simulink library "Simple_lib"  (R2018b)
settings: Solver=ode45  StartTime=0.0  StopTime=10.0  RelTol=1e-3  EnableMultiTasking=on
undefined symbols (not defined in the file or in its folder): Acceptance, beta, C, C_J, C_P, c_wall, dGain, DiscIntNeverNeededParam, Duplex, Electrical_lib, grab, h_fe, i, i3, K_T, Kman, KmanCE, mu_s, n_rev, R_arm, Simplex, systemTs, tau_0, TinIC, Ts, w_0, wallMass, Watch_lib
libraries: $bdroot x407, PlantUtilityBlockset_lib x30, peGeneralControl x22, simulink x11
(part 9 of 14)

== system Simple_lib/Hydraulic/Pump ==
  P : Inport
  w : Inport  Port=2
  T : Inport  Port=3
  Area : Gain
  Area1 : Gain  Gain=-1
  Area3 : Gain  Gain=-1
  Bus Creator : BusCreator  Inputs=2
  Bus Creator1 : BusCreator  Inputs=2
  Bus Selector : BusSelector  OutputSignals=p,T
  Bus Selector1 : BusSelector  OutputSignals=T,p
  PushBack : PlantUtilityBlockset_lib/Utility/Push  SystemSampleTime=-1
  PushBack1 : PlantUtilityBlockset_lib/Utility/Push  SystemSampleTime=-1
  PushBack2 : PlantUtilityBlockset_lib/Utility/Push  SystemSampleTime=-1
  Q : Constant  Value=[100 100 100 100 100 100]
  Q1 : Constant  Value=[100 100 100 100 100 100]
  Sum : Sum  Inputs=+|+
  Terminator : Terminator
  Terminator1 : Terminator
  VolPerRad : Gain
  wires:
  Bus Creator1/1 -> PushBack1/2
  Q1/1 -> Bus Creator1/1  "Q"
  Q/1 -> Bus Creator/2  "Q"
  Bus Creator/1 -> PushBack/2
  Bus Selector1/1 -> Terminator1/1  "<T>"
  PushBack1/1 -> Bus Selector1/1
  PushBack/1 -> Bus Selector/1
  T/1 -> PushBack1/1
  Bus Selector/2 -> Terminator/1  "<T>"
  P/1 -> PushBack/1
  VolPerRad/1 -> Area3/1, Bus Creator1/2  "q"
  Area3/1 -> Bus Creator/1  "q"
  PushBack2/1 -> VolPerRad/1
  Area1/1 -> Sum/2
  Area/1 -> PushBack2/2
  Sum/1 -> Area/1
  Bus Selector1/2 -> Area1/1  "<p>"
  Bus Selector/1 -> Sum/1  "<p>"
  w/1 -> PushBack2/1

== system Simple_lib/Hydraulic/Quadratic Heat Pipe ==
  pT_in : Inport
  Display1 : Display
  Gain : Gain  Gain=-1
  Gain1 : Gain  Gain=1e3
  I1O1BoxIIValveCannelloniHydro6 : Scope
  Product : Product  Inputs=***//  RndMeth=Zero
  Pull : Subsystem  Tag=Electrical  AncestorBlock=PlantUtilityBlockset_lib/Utility/Pull  InitFcn=initDuplex
      mask Display:
      | color('white')
      | plot([0 3], [2 2])
      | plot([0 3], [-2 -2])
      | color('black')
      | 
      | plot([0 1 1], [0 0 0.4])
      | plot([1 1 3], [0.6 1 1])
      | plot([1 3 2 1 0 2], [0.6 0.6 0.4 0.6 0.4 0.4])
      | patch([0 2 1],[0.4 0.4 0.6],[0,0,0])
      | plot([3 2 2], [1 1 0.6])
      | plot([2 2 3], [0.4 -1 -1])
  Push : Subsystem  AncestorBlock=PlantUtilityBlockset_lib/Utility/Push  InitFcn=initSimplex
      mask Display:
      | color('white')
      | plot([0 3], [2 2])
      | plot([0 3], [-2 -2])
      | color('black')
      | 
      | plot([0 2 2 3], [1 1 0 0])
      | plot([1 3 2 1 0 2], [0.6 0.6 0.4 0.6 0.4 0.4])
      | patch([1 3 2],[0.6 0.6 0.4],[0,0,0])
      | plot([0 1 1], [1 1 0.6])
      | plot([1 1 0], [0.4 -1 -1])
  Sign : Signum
  Sum : Sum  Inputs=|++
  area : Gain  Gain=0.1
  area offset : Constant  Value=0.1
  pT_out : Outport
  wires:
  Push/1(OutPot) -> Sum/1
  Sum/1 -> Pull/1(InPot)
  Gain/1 -> Sum/2
  Product/1 -> Gain1/1
  Pull/2(OutFlow) -> Display1/1, I1O1BoxIIValveCannelloniHydro6/1, Product/1, Push/2(InFlow), Sign/1, Product/3
  area offset/1 -> area/1
  Sign/1 -> Product/2
  Gain1/1 -> Gain/1
  area/1 -> Product/5, Product/4
  Pull/1(OutPot) -> pT_out/1
  pT_in/1 -> Push/1(InPot)

== system Simple_lib/Hydraulic/Quadratic Pipe ==
  pT_in : Inport
  Display1 : Display
  Gain : Gain  Gain=-1
  Gain1 : Gain  Gain=1e3
  I1O1BoxIIValveCannelloniHydro6 : Scope
  Product : Product  Inputs=***//  RndMeth=Zero
  Pull : Subsystem  Tag=Electrical  AncestorBlock=PlantUtilityBlockset_lib/Utility/Pull  InitFcn=initDuplex
      mask Display:
      | color('white')
      | plot([0 3], [2 2])
      | plot([0 3], [-2 -2])
      | color('black')
      | 
      | plot([0 1 1], [0 0 0.4])
      | plot([1 1 3], [0.6 1 1])
      | plot([1 3 2 1 0 2], [0.6 0.6 0.4 0.6 0.4 0.4])
      | patch([0 2 1],[0.4 0.4 0.6],[0,0,0])
      | plot([3 2 2], [1 1 0.6])
      | plot([2 2 3], [0.4 -1 -1])
  Push : Subsystem  AncestorBlock=PlantUtilityBlockset_lib/Utility/Push  InitFcn=initSimplex
      mask Display:
      | color('white')
      | plot([0 3], [2 2])
      | plot([0 3], [-2 -2])
      | color('black')
      | 
      | plot([0 2 2 3], [1 1 0 0])
      | plot([1 3 2 1 0 2], [0.6 0.6 0.4 0.6 0.4 0.4])
      | patch([1 3 2],[0.6 0.6 0.4],[0,0,0])
      | plot([0 1 1], [1 1 0.6])
      | plot([1 1 0], [0.4 -1 -1])
  Sign : Signum
  Sum : Sum  Inputs=|++
  area : Gain  Gain=0.1
  area offset : Constant  Value=0.1
  pT_out : Outport
  wires:
  Push/1(OutPot) -> Sum/1
  Sum/1 -> Pull/1(InPot)
  Gain/1 -> Sum/2
  Product/1 -> Gain1/1
  Pull/2(OutFlow) -> Display1/1, I1O1BoxIIValveCannelloniHydro6/1, Product/1, Push/2(InFlow), Sign/1, Product/3
  area offset/1 -> area/1
  Sign/1 -> Product/2
  Gain1/1 -> Gain/1
  area/1 -> Product/5, Product/4
  Pull/1(OutPot) -> pT_out/1
  pT_in/1 -> Push/1(InPot)

== system Simple_lib/Hydraulic/Tank ==
  Ambient Pressure : Constant  Value=1e5
  Duplex : PlantUtilityBlockset_lib/Utility/Pull  Tag=Electrical  SystemSampleTime=-1
  Terminator : Terminator
  Out1 : Outport
  wires:
  Duplex/1 -> Out1/1
  Ambient Pressure/1 -> Duplex/1
  Duplex/2 -> Terminator/1

== system Simple_lib/Hydraulic/Water-Glycol Heat Exchanger ==
  pTSea_in : Inport
  pTGly_in : Inport  Port=2
  Pipe1 : Subsystem  AncestorBlock=PlantUtilityBlockset_lib/Hydraulic/Quadratic Pipe  InitFcn=bond
      mask Display:
      | plot([-1:0.2:1], [1 .7 .5 .4 .35 .32 .35 .4 .5 .7 1])
      | plot([-1:0.2:1], -[1 .7 .5 .4 .35 .32 .35 .4 .5 .7 1])
  Pipe2 : Subsystem  AncestorBlock=PlantUtilityBlockset_lib/Hydraulic/Quadratic Pipe  InitFcn=bond
      mask Display:
      | plot([-1:0.2:1], [1 .7 .5 .4 .35 .32 .35 .4 .5 .7 1])
      | plot([-1:0.2:1], -[1 .7 .5 .4 .35 .32 .35 .4 .5 .7 1])
  pTSea_out : Outport
  pTGly_out : Outport  Port=2
  wires:
  Pipe1/1(pT_out) -> pTSea_out/1
  Pipe2/1(pT_out) -> pTGly_out/1
  pTGly_in/1 -> Pipe2/1(pT_in)
  pTSea_in/1 -> Pipe1/1(pT_in)

== system Simple_lib/Hydraulic/X Heat Exchanger ==
  in1 : Inport
  in2 : Inport  Port=2
  Pipe1 : Subsystem  AncestorBlock=PlantUtilityBlockset_lib/Hydraulic/Quadratic Pipe
      mask Display:
      | plot([-1:0.2:1], [1 .7 .5 .4 .35 .32 .35 .4 .5 .7 1])
      | plot([-1:0.2:1], -[1 .7 .5 .4 .35 .32 .35 .4 .5 .7 1])
  Pipe2 : Subsystem  AncestorBlock=PlantUtilityBlockset_lib/Hydraulic/Quadratic Pipe
      mask Display:
      | plot([-1:0.2:1], [1 .7 .5 .4 .35 .32 .35 .4 .5 .7 1])
      | plot([-1:0.2:1], -[1 .7 .5 .4 .35 .32 .35 .4 .5 .7 1])
  out1 : Outport
  out2 : Outport  Port=2
  wires:
  Pipe1/1(pT_out) -> out1/1
  Pipe2/1(pT_out) -> out2/1
  in2/1 -> Pipe2/1(pT_in)
  in1/1 -> Pipe1/1(pT_in)

== system Simple_lib/Junkyard/CinWall ==
  C : Subsystem  AncestorBlock=PlantUtilityBlockset_lib/Electrical/C  mask{C=wallMass*c_wall}
      mask prompts: C "Capacitance"
      mask Display:
      | color('white')
      | plot([-1 1 1 -1 -1], [-1 -1 1 1 -1])
      | color('black')
      | plot([1.0 1.8 1.8 1.0], [0 .1 -.1 0])
      | plot([-1 -1], [-1 1])
      | plot([1 1], [-1 1])
  Gnd : Subsystem  AncestorBlock=PlantUtilityBlockset_lib/Electrical/Gnd
      mask Display:
      | color('white')
      | plot([-1 1 1 -1 -1], [-1 -1 1 1 -1])
      | 
      | color('black')
      | plot([1.0 1.18 1.18 1.0], [0 .15 -.15 0])
      | 
      | plot([-0.4 -0.4],[-1 1])
      | plot([-0.6 -0.6], [-0.6 0.6])
      | plot([-0.8 -0.8],[-0.2 0.2])
      | 
      | plot([-0.4 1],[0 0])
  Out1 : Outport
  wires:
  C/1(Out1) -> Out1/1
  Gnd/1(Out1) -> C/1(In1)

== system Simple_lib/Junkyard/Conventional Flow  ==
  In1 : Inport
  Out1 : Outport
  wires:
  In1/1 -> Out1/1

== system Simple_lib/Junkyard/R13 ==
  In1 : Inport
  Duplex : Subsystem  Tag=Electrical  AncestorBlock=PlantUtilityBlockset_lib/Utility/Duplex  InitFcn=initDuplex
      mask Display:
      | color('white')
      | plot([0 3], [2 2])
      | plot([0 3], [-2 -2])
      | color('black')
      | 
      | plot([0 1 1], [0 0 0.4])
      | plot([1 1 3], [0.6 1 1])
      | plot([1 3 2 1 0 2], [0.6 0.6 0.4 0.6 0.4 0.4])
      | patch([0 2 1],[0.4 0.4 0.6],[0,0,0])
      | plot([3 2 2], [1 1 0.6])
      | plot([2 2 3], [0.4 -1 -1])
  Simplex : Subsystem  Tag=Electrical  AncestorBlock=PlantUtilityBlockset_lib/Utility/Simplex  InitFcn=initSimplex
      mask Display:
      | color('white')
      | plot([0 3], [2 2])
      | plot([0 3], [-2 -2])
      | color('black')
      | 
      | plot([0 2 2 3], [1 1 0 0])
      | plot([1 3 2 1 0 2], [0.6 0.6 0.4 0.6 0.4 0.4])
      | patch([1 3 2],[0.6 0.6 0.4],[0,0,0])
      | plot([0 1 1], [1 1 0.6])
      | plot([1 1 0], [0.4 -1 -1])
  Sum : Sum  Inputs=|++
  resistance : Gain  Gain=R
  Out1 : Outport
  wires:
  In1/1 -> Simplex/1(InPot)
  Duplex/1(OutPot) -> Out1/1
  Duplex/2(OutFlow) -> Simplex/2(InFlow), resistance/1
  Simplex/1(OutPot) -> Sum/1
  resistance/1 -> Sum/2
  Sum/1 -> Duplex/1(InPot)

== system Simple_lib/Junkyard/R17 ==
  In1 : Inport
  In2 : Inport  Port=2
  1/R1 : Gain  Gain=-1
  1/R2 : Gain  Gain=-1
  Discrete-Time Integrator1 : DiscreteIntegrator  gainval=1/10/Ts  SampleTime=Ts  ICPrevOutput=DiscIntNeverNeededParam  ICPrevScaledInput=DiscIntNeverNeededParam
  Simplex : Subsystem  Tag=Electrical  AncestorBlock=PlantUtilityBlockset_lib/Utility/Simplex  InitFcn=initSimplex
      mask Display:
      | color('white')
      | plot([0 3], [2 2])
      | plot([0 3], [-2 -2])
      | color('black')
      | 
      | plot([0 2 2 3], [1 1 0 0])
      | plot([1 3 2 1 0 2], [0.6 0.6 0.4 0.6 0.4 0.4])
      | patch([1 3 2],[0.6 0.6 0.4],[0,0,0])
      | plot([0 1 1], [1 1 0.6])
      | plot([1 1 0], [0.4 -1 -1])
  Simplex1 : Subsystem  Tag=Electrical  AncestorBlock=PlantUtilityBlockset_lib/Utility/Simplex  InitFcn=initSimplex
      mask Display:
      | color('white')
      | plot([0 3], [2 2])
      | plot([0 3], [-2 -2])
      | color('black')
      | 
      | plot([0 2 2 3], [1 1 0 0])
      | plot([1 3 2 1 0 2], [0.6 0.6 0.4 0.6 0.4 0.4])
      | patch([1 3 2],[0.6 0.6 0.4],[0,0,0])
      | plot([0 1 1], [1 1 0.6])
      | plot([1 1 0], [0.4 -1 -1])
  Sum : Sum  Inputs=+|+
  Sum1 : Sum  Inputs=|+-
  conductance : Gain  Gain=1/R
  wires:
  Discrete-Time Integrator1/1 -> Sum1/2, 1/R1/1, Simplex/2(InFlow)
  Sum1/1 -> Discrete-Time Integrator1/1
  1/R1/1 -> Simplex1/2(InFlow)
  Simplex1/1(OutPot) -> Sum/2
  In2/1 -> Simplex1/1(InPot)
  Sum/1 -> conductance/1
  1/R2/1 -> Sum/1
  Simplex/1(OutPot) -> 1/R2/1
  In1/1 -> Simplex/1(InPot)
  conductance/1 -> Sum1/1

== system Simple_lib/Junkyard/ThermoMeter ==
  In : Inport
  Ground : Ground
  PushBack : Subsystem  AncestorBlock=PlantUtilityBlockset_lib/Utility/Push  InitFcn=initSimplex
      mask Display:
      | color('white')
      | plot([0 3], [2 2])
      | plot([0 3], [-2 -2])
      | color('black')
      | 
      | plot([0 2 2 3], [1 1 0 0])
      | plot([1 3 2 1 0 2], [0.6 0.6 0.4 0.6 0.4 0.4])
      | patch([1 3 2],[0.6 0.6 0.4],[0,0,0])
      | plot([0 1 1], [1 1 0.6])
      | plot([1 1 0], [0.4 -1 -1])
  T : Outport
  wires:
  In/1 -> PushBack/1(InPot)
  PushBack/1(OutPot) -> T/1
  Ground/1 -> PushBack/2(InFlow)

== system Simple_lib/Junkyard/Unconventional Flow ==
  In1 : Inport
  Out1 : Outport
  wires:
  In1/1 -> Out1/1

== system Simple_lib/Magnetic/BiGain ==
  In1 : Inport
  Bus Creator1 : BusCreator  Inputs=2
  Bus Selector : BusSelector  OutputSignals=F,M
  _in : $bdroot/Translational/_in  Level=v  Flow=F
  _out : $bdroot/Translational/_out  Tag=Electrical  Level=v  Flow=F
  k_flow : Gain  Gain=k_flow
  k_flow1 : Gain  Gain=k_flow
  k_flow2 : Gain  Gain=k_flow
  k_level : Gain  Gain=k_level
  Out1 : Outport
  wires:
  _out/1 -> Out1/1
  _in/1 -> k_level/1
  In1/1 -> _in/1
  k_level/1 -> _out/1
  _out/2 -> Bus Selector/1
  k_flow/1 -> Bus Creator1/1  "F"
  Bus Selector/2 -> k_flow2/1  "<M>"
  Bus Selector/1 -> k_flow/1  "<F>"
  Bus Creator1/1 -> _in/2
  k_flow2/1 -> k_flow1/1  "M"
  k_flow1/1 -> Bus Creator1/2  "M"

== system Simple_lib/Magnetic/Core ==
  + : Inport
  - : Inport  Port=2
  1/R3 : Gain  Gain=-1
  Bus Creator : BusCreator  Inputs=2
  Bus Creator1 : BusCreator  Inputs=2
  Derivative : Derivative
  Ground : Ground
  Ground1 : Ground
  M : Gain  Gain=b
  Sum : Sum  Inputs=+|-
  _neg : $bdroot/Magnetic/_in  Level=MMF  Flow=Phi
  _pos : $bdroot/Magnetic/_in  Level=MMF  Flow=Phi
  wires:
  1/R3/1 -> Bus Creator/1  "dPhi"
  Sum/1 -> Derivative/1
  Derivative/1 -> M/1  "dI1"
  -/1 -> _neg/1
  _pos/1 -> Sum/1  "I1"
  _neg/1 -> Sum/2  "I2"
  M/1 -> 1/R3/1, Bus Creator1/1  "dPhi"
  Bus Creator1/1 -> _pos/2
  Ground/1 -> Bus Creator/2  "MagneticInertia"
  +/1 -> _pos/1  "mmf"
  Bus Creator/1 -> _neg/2
  Ground1/1 -> Bus Creator1/2  "MagneticInertia"

== system Simple_lib/Magnetic/Core_old ==
  + : Inport
  - : Inport  Port=2
  1/R1 : Gain  Gain=b
  1/R3 : Gain  Gain=b
  Bus Creator : BusCreator  Inputs=2
  Bus Creator1 : BusCreator  Inputs=2
  Discrete Derivative : simulink/Discrete/Discrete Derivative  gainval=1  ICPrevScaledInput=0.0  OutMin=[]  OutMax=[]  OutDataType=fixdt(1, 16)  OutScaling=2^-10  DoSatur=off
  Discrete Derivative1 : simulink/Discrete/Discrete Derivative  gainval=1  ICPrevScaledInput=0.0  OutMin=[]  OutMax=[]  OutDataType=fixdt(1, 16)  OutScaling=2^-10  DoSatur=off
  Ground : Ground
  Ground1 : Ground
  _neg : $bdroot/Magnetic/_in  Level=MMF  Flow=Phi
  _pos : $bdroot/Magnetic/_in  Level=MMF  Flow=Phi
  wires:
  Discrete Derivative1/1 -> 1/R1/1  "dI1"
  Discrete Derivative/1 -> 1/R3/1  "dI2"
  -/1 -> _neg/1
  1/R1/1 -> Bus Creator/1  "dPhi"
  _pos/1 -> Discrete Derivative1/1  "I1"
  _neg/1 -> Discrete Derivative/1  "I2"
  1/R3/1 -> Bus Creator1/1  "dPhi"
  Bus Creator1/1 -> _pos/2
  Ground/1 -> Bus Creator/2  "MagneticInertia"
  +/1 -> _pos/1  "mmf"
  Bus Creator/1 -> _neg/2
  Ground1/1 -> Bus Creator1/2  "MagneticInertia"

== system Simple_lib/Magnetic/Friction ==
  pos : Inport
  K : Inport  Port=2
  neg : Inport  Port=3
  1/R1 : Gain  Gain=-1
  1/R2 : Gain  Gain=-1
  1/R3 : Gain  Gain=-1
  Bus Creator : BusCreator  Inputs=2
  Bus Creator1 : BusCreator  Inputs=2
  Discrete-Time Integrator : DiscreteIntegrator  gainval=1  SampleTime=-1  ICPrevOutput=DiscIntNeverNeededParam  ICPrevScaledInput=DiscIntNeverNeededParam
  Exp : Math  SaturateOnIntegerOverflow=on
  Gain : Gain  Gain=-1/2
  Ground : Ground
  Multiply : Product
  Multiply1 : Product  Inputs=**//
  Multiply2 : Product  Inputs=**/
  Sum : Sum  Inputs=+|+
  Sum1 : Sum  Inputs=|++
  _neg : $bdroot/Translational/_in  Level=v  Flow=F
  _pos : $bdroot/Translational/_in  Level=v  Flow=F
  friction : Trigonometry  Operator=tanh
  grab : Gain  Gain=grab
  sigma : Constant  Value=s
  synche : Gain  Gain=Ki/sqrt(2*pi)
  wires:
  synche/1 -> Sum1/2
  friction/1 -> Multiply/2
  Sum/1 -> grab/1
  Discrete-Time Integrator/1 -> synche/1
  Sum1/1 -> friction/1
  Gain/1 -> Exp/1
  sigma/1 -> Multiply1/3, Multiply1/4, Multiply2/3
  Multiply2/1 -> Discrete-Time Integrator/1
  Exp/1 -> Multiply2/2
  Multiply1/1 -> Gain/1
  _neg/1 -> 1/R3/1
  Multiply/1 -> 1/R2/1
  _pos/1 -> Sum/1
  grab/1 -> Multiply2/1, Multiply1/2, Multiply1/1, Sum1/1
  pos/1 -> _pos/1
  neg/1 -> _neg/1
  K/1 -> Multiply/1
  Bus Creator1/1 -> _pos/2
  1/R2/1 -> Bus Creator1/1, 1/R1/1  "F"
  Bus Creator/1 -> _neg/2
  Ground/1 -> Bus Creator1/2, Bus Creator/2  "M"
  1/R1/1 -> Bus Creator/1  "F"
  1/R3/1 -> Sum/2

== system Simple_lib/Magnetic/Sink ==
  In1 : Inport
  Bus Creator : BusCreator  Inputs=2
  Constant : Constant  Value=m
  Ground : Ground
  Terminator : Terminator
  _at : $bdroot/Translational/_in  Level=v  Flow=F
  wires:
  Bus Creator/1 -> _at/2
  In1/1 -> _at/1
  _at/1 -> Terminator/1
  Ground/1 -> Bus Creator/1  "F"
  Constant/1 -> Bus Creator/2  "M"

== system Simple_lib/Magnetic/Source ==
  note: Newton's law for all the applied torques (real parts) and the inertials (imaginary parts).
  Bus Selector : BusSelector  OutputSignals=F,M
  Constant : Constant  Value=m
  Discrete-Time Integrator1 : DiscreteIntegrator  gainval=1  InitialCondition=v_0  SampleTime=-1  ICPrevOutput=DiscIntNeverNeededParam  ICPrevScaledInput=DiscIntNeverNeededParam
  Multiply : Product  Inputs=*/
  Saturation : Saturate  UpperLimit=inf  LowerLimit=Ts*1e-3
  Sum : Sum  Inputs=|++
  _at : $bdroot/Translational/_out  Tag=Electrical  Level=v  Flow=F
  Out1 : Outport
  wires:
  _at/1 -> Out1/1
  Multiply/1 -> Discrete-Time Integrator1/1
  _at/2 -> Bus Selector/1
  Bus Selector/1 -> Multiply/1  "<F>"
  Bus Selector/2 -> Sum/1  "<M>"
  Sum/1 -> Saturation/1
  Constant/1 -> Sum/2
  Discrete-Time Integrator1/1 -> _at/1
  Saturation/1 -> Multiply/2

== system Simple_lib/Magnetic/SpringDamper ==
  in : Inport
  Damping : $bdroot/Translational/Damping  b=b_damper
  Source1 : $bdroot/Translational/Source  m=m_out  v_0=v_0
      settings: AttributesFormatString=%<m> kg
  Stiffness : $bdroot/Translational/Stiffness  k_spring=k_spring  s_0=s_0  I_spring=m_split  b_series=b_spring
  Terminator : Terminator
  out : Outport
  wires:
  in/1 -> Damping/1, Stiffness/1
  Source1/1 -> Damping/2, Stiffness/2, out/1
  Stiffness/1 -> Terminator/1

== system Simple_lib/Magnetic/Stiffness ==
  + : Inport
  - : Inport  Port=2
  Bus Creator : BusCreator  Inputs=2
  Bus Creator1 : BusCreator  Inputs=2
  Constant : Constant  Value=I_spring/2
  Constant1 : Constant  Value=I_spring/2
  Discrete-Time Integrator1 : DiscreteIntegrator  gainval=1  InitialCondition=s_0  SampleTime=-1  ICPrevOutput=DiscIntNeverNeededParam  ICPrevScaledInput=DiscIntNeverNeededParam
  Gain : Gain  Gain=-k_spring
  Gain1 : Gain  Gain=k_spring
  Gain2 : Gain  Gain=2/b_series
  Gain3 : Gain  Gain=2/b_series
  Sum : Sum  Inputs=+|-
  Sum1 : Sum  Inputs=++|
  Sum2 : Sum  Inputs=++|
  _neg : $bdroot/Translational/_in  Level=v  Flow=F
  _pos : $bdroot/Translational/_in  Level=v  Flow=F
  cmp : Outport
  wires:
  _neg/1 -> Sum2/1
  -/1 -> _neg/1
  Sum/1 -> Discrete-Time Integrator1/1
  _pos/1 -> Sum1/1
  +/1 -> _pos/1
  Bus Creator1/1 -> _pos/2
  Bus Creator/1 -> _neg/2
  Discrete-Time Integrator1/1 -> cmp/1, Gain1/1, Gain/1  "cmp"
  Constant/1 -> Bus Creator1/2  "M"
  Constant1/1 -> Bus Creator/1  "M"
  Sum2/1 -> Sum/2
  Sum1/1 -> Sum/1
  Gain/1 -> Gain2/1, Bus Creator1/1  "F"
  Gain1/1 -> Bus Creator/2, Gain3/1  "F"
  Gain2/1 -> Sum1/2
  Gain3/1 -> Sum2/2

== system Simple_lib/Magnetic/_in ==
  note: {\bf\_in - wraps up the {\itInflow} block}
      |
      | The init function {\itinit_in} sets up the logging of the level and flow names.
  in : Inport
  back : Inport  Port=2
  Bus Selector : BusSelector  OutputSignals=dPhi,MagneticInertia
  Inflow : $bdroot/Utility/Inflow  SystemSampleTime=-1
  Mux : Mux  Inputs=2
  out : Outport
  wires:
  in/1 -> Inflow/1  "MMF"
  back/1 -> Bus Selector/1
  Bus Selector/2 -> Mux/2  "<MagneticInertia>"
  Bus Selector/1 -> Mux/1  "<dPhi>"
  Inflow/1 -> out/1
  Mux/1 -> Inflow/2

== system Simple_lib/Magnetic/_out ==
  note: {\bf\_out - buses out and logs the signals from the generic {\itOutflow} block}
      |
      | The init function {\itinit\_out} sets up the logging.
  in : Inport  Tag=NOFLUX
  Bus Creator : BusCreator  Inputs=2
  Constant : Constant  Value=[0;0]
  Demux : Demux  Outputs=2
  Outflow : $bdroot/Utility/Outflow  Tag=Electrical  SystemSampleTime=-1
  Sum : Sum  Inputs=|++
  Sum1 : Sum  Inputs=+  CollapseMode=Specified dimension  CollapseDim=2
  out : Outport
  backs : Outport  Tag=NOFLUX  Port=2
  wires:
  Outflow/1 -> out/1
  Sum1/1 -> Sum/1
  Demux/1 -> Bus Creator/1  "dPhi"
  Bus Creator/1 -> backs/1
  Outflow/2 -> Sum1/1
  in/1 -> Outflow/1  "MMF"
  Demux/2 -> Bus Creator/2  "MagneticInertia"
  Constant/1 -> Sum/2
  Sum/1 -> Demux/1

== system Simple_lib/Magnetic/magR ==
  + : Inport
  - : Inport  Port=2
  1/R3 : Gain  Gain=b
  Bus Creator : BusCreator  Inputs=2
  Bus Creator1 : BusCreator  Inputs=2
  Discrete Derivative : simulink/Discrete/Discrete Derivative  Commented=through  gainval=1  ICPrevScaledInput=0.0  OutMin=[]  OutMax=[]  OutDataType=fixdt(1, 16)  OutScaling=2^-10  DoSatur=off
  Gain1 : Gain  Gain=-1
  Ground : Ground
  Ground1 : Ground
  Sum : Sum  Inputs=+|-
  _neg : $bdroot/Magnetic/_in  Level=MMF  Flow=Phi
  _pos : $bdroot/Magnetic/_in  Level=MMF  Flow=Phi
  wires:
  Discrete Derivative/1 -> 1/R3/1
  -/1 -> _neg/1
  _neg/1 -> Sum/2
  1/R3/1 -> Bus Creator/1, Gain1/1  "dPhi"
  Bus Creator1/1 -> _pos/2
  Ground/1 -> Bus Creator/2  "MagneticInertia"
  +/1 -> _pos/1  "mmf"
  _pos/1 -> Sum/1
  Sum/1 -> Discrete Derivative/1
  Bus Creator/1 -> _neg/2
  Ground1/1 -> Bus Creator1/2  "MagneticInertia"
  Gain1/1 -> Bus Creator1/1  "dPhi"

== system Simple_lib/Rotational/BiGain ==
  In1 : Inport
  Bus Creator1 : BusCreator  Inputs=3
  Bus Selector : BusSelector  OutputSignals=tau,c,J
  _in : $bdroot/Rotational/_in  Level=w  Flow=tau
  _out : $bdroot/Rotational/_out  Tag=Electrical  Level=w  Flow=tau
  k_flow{1..5} (5 alike) : Gain  Gain=k_flow
  k_pot : Gain  Gain=k_flow
  Out1 : Outport
  wires:
  _out/1 -> Out1/1
  _in/1 -> k_pot/1
  In1/1 -> _in/1
  Bus Creator1/1 -> _in/2
  k_pot/1 -> _out/1
  _out/2 -> Bus Selector/1
  Bus Selector/1 -> k_flow1/1  "<tau>"
  Bus Selector/3 -> k_flow3/1  "<J>"
  k_flow1/1 -> Bus Creator1/1  "tau"
  k_flow2/1 -> Bus Creator1/3  "J"
  k_flow3/1 -> k_flow2/1  "M"
  Bus Selector/2 -> k_flow5/1  "<c>"
  k_flow4/1 -> Bus Creator1/2  "c"
  k_flow5/1 -> k_flow4/1

== system Simple_lib/Rotational/Damping ==
  + : Inport
  - : Inport  Port=2
  1/R3 : Gain  Gain=b
  Bus Creator : BusCreator  Inputs=3
  Bus Creator1 : BusCreator  Inputs=3
  Constant : Constant  Value=b
  Gain1 : Gain  Gain=-1
  Gain2 : Gain  Gain=-1
  Ground : Ground
  Sum : Sum  Inputs=+|+
  _neg : $bdroot/Rotational/_in  Level=w  Flow=tau
  _pos : $bdroot/Rotational/_in  Level=w  Flow=tau
  wires:
  Constant/1 -> Bus Creator1/2, Bus Creator/2  "c"
  _neg/1 -> Gain2/1
  1/R3/1 -> Bus Creator1/1, Gain1/1  "tau"
  Bus Creator1/1 -> _pos/2
  +/1 -> _pos/1
  _pos/1 -> Sum/1
  Sum/1 -> 1/R3/1
  -/1 -> _neg/1
  Bus Creator/1 -> _neg/2
  Ground/1 -> Bus Creator1/3, Bus Creator/1  "J"
  Gain1/1 -> Bus Creator/3  "tau"
  Gain2/1 -> Sum/2  "tau"

== system Simple_lib/Rotational/Friction ==
  pos : Inport
  K : Inport  Port=2
  neg : Inport  Port=3
  1/R1 : Gain  Gain=-1
  Bus Creator : BusCreator  Inputs=3
  Bus Creator1 : BusCreator  Inputs=3
  Calculate Slip : Subsystem
  Derivative : Subsystem
  Gaussian Spring : Subsystem
  Ground : Ground
  Multiply : Product
  Sum1 : Sum  Inputs=|++
  _neg : $bdroot/Rotational/_in  Level=w  Flow=tau
  _pos : $bdroot/Rotational/_in  Level=w  Flow=tau
  wires:
  _neg/1 -> Calculate Slip/2(w_neg)  "w_neg"
  _pos/1 -> Calculate Slip/1(w_pos)  "w_pos"
  Calculate Slip/1(slip) -> Derivative/2(x), Gaussian Spring/1(slip), Sum1/1
  Derivative/1(dy/dx) -> Bus Creator1/2, Bus Creator/2  "c"
  Gaussian Spring/1(tau) -> Sum1/2
  1/R1/1 -> Bus Creator1/3  "tau"
  Sum1/1 -> Multiply/2
  neg/1 -> _neg/1
  pos/1 -> _pos/1
  K/1 -> Multiply/1
  Bus Creator1/1 -> _neg/2
  Multiply/1 -> Derivative/1(y), Bus Creator/1, 1/R1/1  "tau"
  Bus Creator/1 -> _pos/2
  Ground/1 -> Bus Creator1/1, Bus Creator/3  "J"

== system Simple_lib/Rotational/Inertia ==
  In1 : Inport
  Bus Creator : BusCreator  Inputs=3
  Constant : Constant  Value=I
  Ground : Ground
  Ground1 : Ground
  Terminator : Terminator
  _at : $bdroot/Rotational/_in  Level=w  Flow=tau
  wires:
  Ground1/1 -> Bus Creator/2  "c"
  Bus Creator/1 -> _at/2
  In1/1 -> _at/1
  _at/1 -> Terminator/1
  Ground/1 -> Bus Creator/1  "tau"
  Constant/1 -> Bus Creator/3  "J"

== system Simple_lib/Rotational/Lump ==
  note: Newton's law for all the applied torques and the inertials.
      | If the inertia sum is too small to give sensible results we approximate from the damping coefficients.
      | If that is really small we saturate at J = e-12 Nm2.
      | We also saturate the overall acceleration to configurable parameter max_accel.
  Abs2 : Abs
  Abs3 : Abs
  Bus Selector : BusSelector  OutputSignals=tau,c,J
  Constant : Constant  Value=w_0
  Constant1 : Constant  Value=1/2
  Ground : Ground
  Integrator (Discrete or Continuous) : peGeneralControl/Integrator (Discrete or Continuous)  LabelModeActiveChoice=Discrete  ExternalReset=level  LimitType=Anti-windup  B=inf  A=-inf  Ts=-1
  Max1 : MinMax  Function=max  Inputs=2
  Momentum outflow decelerates : Gain  Gain=-1
  Multiply : Product  Inputs=*/
  Multiply1 : Product  Inputs=3
  Multiply2 : Product
  Saturation : Saturate  UpperLimit=inf  LowerLimit=1e-12
      settings: AttributesFormatString=|
      | %<UpperLimit>
      | %<LowerLimit>
  Saturation3 : Saturate  UpperLimit=max_accel  LowerLimit=-max_accel
      settings: AttributesFormatString=|
      | %<UpperLimit>
      | %<LowerLimit>
  Terminator : Terminator
  Terminator1 : Terminator
  Weighted Sample Time1 : SampleTimeMath  TsampMathOp=*  weightValue=1
  _off : $bdroot/Rotational/_out  Tag=Electrical  Level=w  Flow=tau
  Out1 : Outport
  wires:
  Constant1/1 -> Multiply1/2
  Multiply1/1 -> Terminator1/1  "energy"
  Multiply2/1 -> Terminator/1, Multiply1/3  "conserved_quantity"
  Saturation3/1 -> Integrator (Discrete or Continuous)/1  "dw_sat"
  Abs3/1 -> Max1/1  "JestPos"
  Abs2/1 -> Max1/2  "Jpos"
  Bus Selector/2 -> Weighted Sample Time1/1  "<c>"
  Max1/1 -> Saturation/1  "Jeff"
  Weighted Sample Time1/1 -> Abs3/1  "Jest"
  _off/1 -> Out1/1
  Multiply/1 -> Saturation3/1  "dw"
  _off/2 -> Bus Selector/1
  Bus Selector/1 -> Momentum outflow decelerates/1  "<tau>"
  Bus Selector/3 -> Abs2/1  "<J>"
  Integrator (Discrete or Continuous)/1 -> _off/1, Multiply1/1, Multiply2/1  "w"
  Saturation/1 -> Multiply/2, Multiply2/2  "Jeff_sat"
  Constant/1 -> Integrator (Discrete or Continuous)/3
  Ground/1 -> Integrator (Discrete or Continuous)/2
  Momentum outflow decelerates/1 -> Multiply/1

== system Simple_lib/Rotational/M1 ==
  In1 : Inport
  _at : $bdroot/Rotational/_out  Tag=Electrical  Level=w  Flow=tau
  _thru : $bdroot/Rotational/_in  Level=w  Flow=tau
  Out1 : Outport
  wires:
  _at/1 -> Out1/1
  In1/1 -> _thru/1
  _thru/1 -> _at/1
  _at/2 -> _thru/2

== system Simple_lib/Rotational/NonLinear Compliance ==
  + : Inport
  - : Inport  Port=2
  1-D Lookup Table : Lookup_n-D  NumberOfTableDimensions=1  BreakpointsForDimension1=[-5:5]*10  Table=[100 10 1 0 0 0 0 0 1 10 100]  InternalRulePriority=Speed  RndMeth=Simplest  InputSameDT=on
  Bus Creator : BusCreator  Inputs=2
  Bus Creator1 : BusCreator  Inputs=2
  Constant : Constant  Value=I_spring/2
  Constant1 : Constant  Value=I_spring/2
  Discrete-Time Integrator1 : DiscreteIntegrator  gainval=1  InitialCondition=theta_0  SampleTime=-1  ICPrevOutput=DiscIntNeverNeededParam  ICPrevScaledInput=DiscIntNeverNeededParam
  Gain : Gain  Gain=-k_spring
  Gain1 : Gain  Gain=k_spring
  Gain2 : Gain  Gain=2/b_series
  Gain3 : Gain  Gain=2/b_series
  Gain4 : Gain  Gain=-1
  Sum : Sum  Inputs=+|-
  Sum1 : Sum  Inputs=++|
  Sum2 : Sum  Inputs=++|
  _neg : $bdroot/Rotational/_in  Level=w  Flow=tau
  _pos : $bdroot/Rotational/_in  Level=w  Flow=tau
  cmp : Outport
  wires:
  Gain4/1 -> cmp/1, Gain/1, Gain1/1
  1-D Lookup Table/1 -> Gain4/1
  _neg/1 -> Sum2/1
  -/1 -> _neg/1
  Sum/1 -> Discrete-Time Integrator1/1
  _pos/1 -> Sum1/1
  +/1 -> _pos/1
  Bus Creator1/1 -> _pos/2
  Bus Creator/1 -> _neg/2
  Discrete-Time Integrator1/1 -> 1-D Lookup Table/1  "cmp"
  Constant/1 -> Bus Creator1/2  "J"
  Constant1/1 -> Bus Creator/1  "J"
  Sum2/1 -> Sum/2
  Sum1/1 -> Sum/1
  Gain/1 -> Gain2/1, Bus Creator1/1  "tau"
  Gain1/1 -> Bus Creator/2, Gain3/1  "tau"
  Gain2/1 -> Sum1/2
  Gain3/1 -> Sum2/2

== system Simple_lib/Rotational/Power ==
  " " : Inport
  Bus Creator1 : BusCreator  Inputs=2
  Bus Selector : BusSelector  OutputSignals=tau,J
  Multiply : Product
  Torque_Speed : simulink/Sinks/XY Graph  Commented=on  xmin=0  xmax=200  ymin=-1  ymax=1  st=-1
  _in : $bdroot/Rotational/_in  Level=w  Flow=tau
  _out : $bdroot/Rotational/_out  Tag=Electrical  Level=w  Flow=tau
  "  " : Outport
  > : Outport  Port=2
  wires:
  Multiply/1 -> >/1
  _out/1 -> "  "/1
  " "/1 -> _in/1
  Bus Creator1/1 -> _in/2
  _in/1 -> Torque_Speed/1, _out/1, Multiply/1  "w"
  _out/2 -> Bus Selector/1
  Bus Selector/1 -> Bus Creator1/1, Torque_Speed/2, Multiply/2  "<tau>"
  Bus Selector/2 -> Bus Creator1/2  "<J>"

== system Simple_lib/Rotational/Speed ==
  w : Inport
  Terminator1 : Terminator
  _at : $bdroot/Rotational/_out  Tag=Electrical  Level=w  Flow=tau
  sys : Outport
  wires:
  w/1 -> _at/1
  _at/1 -> sys/1
  _at/2 -> Terminator1/1

== system Simple_lib/Rotational/SpringDamper ==
  in : Inport
  Damping : $bdroot/Rotational/Damping  b=b_damper
  Source : $bdroot/Rotational/Lump  w_0=w_0  max_accel=inf
  Stiffness : $bdroot/Rotational/Stiffness  k_spring=k_spring  theta_0=theta_0  I_spring=I_split  b_series=b_spring
  Terminator : Terminator
  out : Outport
  wires:
  in/1 -> Stiffness/1, Damping/1
  Source/1 -> Stiffness/2, Damping/2, out/1
  Stiffness/1 -> Terminator/1

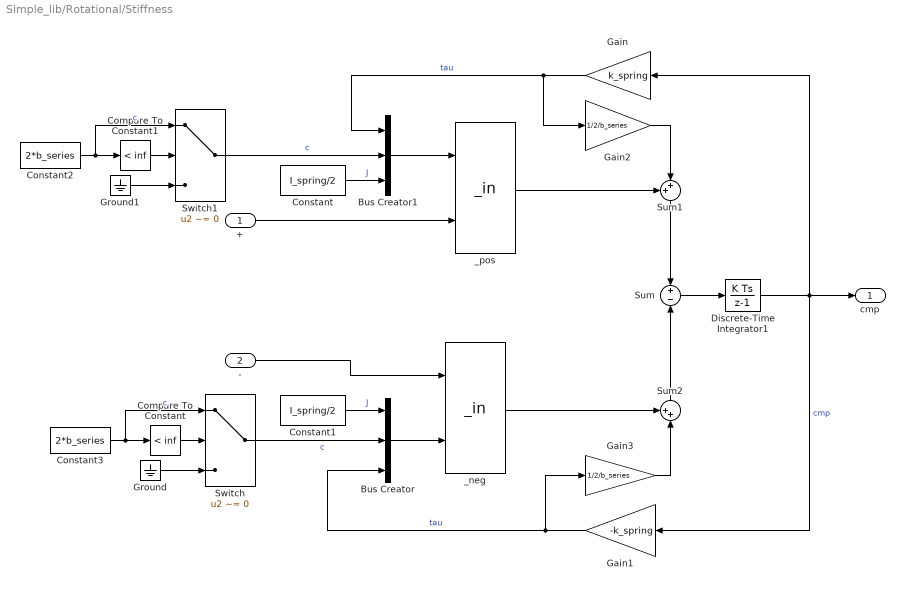
== system Simple_lib/Rotational/Stiffness ==
  + : Inport
  - : Inport  Port=2
  Bus Creator : BusCreator  Inputs=3
  Bus Creator1 : BusCreator  Inputs=3
  Compare To Constant : simulink/Logic and Bit Operations/Compare To Constant  relop=<  const=inf  OutDataTypeStr=boolean
  Compare To Constant1 : simulink/Logic and Bit Operations/Compare To Constant  relop=<  const=inf  OutDataTypeStr=boolean
  Constant : Constant  Value=I_spring/2
  Constant1 : Constant  Value=I_spring/2
  Constant2 : Constant  Value=2*b_series
  Constant3 : Constant  Value=2*b_series
  Discrete-Time Integrator1 : DiscreteIntegrator  gainval=1  InitialCondition=theta_0  SampleTime=-1  ICPrevOutput=DiscIntNeverNeededParam  ICPrevScaledInput=DiscIntNeverNeededParam
  Gain : Gain  Gain=k_spring
  Gain1 : Gain  Gain=-k_spring
  Gain2 : Gain  Gain=1/2/b_series
  Gain3 : Gain  Gain=1/2/b_series
  Ground : Ground
  Ground1 : Ground
  Sum : Sum  Inputs=+|-
  Sum1 : Sum  Inputs=++|
  Sum2 : Sum  Inputs=++|
  Switch : Switch  Criteria=u2 ~= 0
  Switch1 : Switch  Criteria=u2 ~= 0
  _neg : $bdroot/Rotational/_in  Level=w  Flow=tau
  _pos : $bdroot/Rotational/_in  Level=w  Flow=tau
  cmp : Outport
  wires:
  Constant3/1 -> Switch/1, Compare To Constant/1  "c"
  Switch1/1 -> Bus Creator1/2  "c"
  _neg/1 -> Sum2/1
  -/1 -> _neg/1
  Sum/1 -> Discrete-Time Integrator1/1
  _pos/1 -> Sum1/1
  +/1 -> _pos/1
  Bus Creator1/1 -> _pos/2
  Bus Creator/1 -> _neg/2
  Discrete-Time Integrator1/1 -> cmp/1, Gain1/1, Gain/1  "cmp"
  Constant/1 -> Bus Creator1/3  "J"
  Constant1/1 -> Bus Creator/1  "J"
  Sum2/1 -> Sum/2
  Sum1/1 -> Sum/1
  Gain/1 -> Gain2/1, Bus Creator1/1  "tau"
  Gain1/1 -> Bus Creator/3, Gain3/1  "tau"
  Gain2/1 -> Sum1/2
  Gain3/1 -> Sum2/2
  Compare To Constant/1 -> Switch/2
  Ground/1 -> Switch/3
  Switch/1 -> Bus Creator/2  "c"
  Ground1/1 -> Switch1/3
  Compare To Constant1/1 -> Switch1/2
  Constant2/1 -> Switch1/1, Compare To Constant1/1  "c"

== system Simple_lib/Rotational/Torque ==
  sys : Inport
  tau : Inport  Port=2
  Bus Creator : BusCreator  Inputs=3
  Ground : Ground
  Ground1 : Ground
  Terminator1 : Terminator
  _at : $bdroot/Rotational/_in  Level=w  Flow=tau
  wires:
  tau/1 -> Bus Creator/1  "tau"
  _at/1 -> Terminator1/1
  sys/1 -> _at/1
  Bus Creator/1 -> _at/2
  Ground/1 -> Bus Creator/3  "J"
  Ground1/1 -> Bus Creator/2  "c"

== system Simple_lib/Rotational/_in ==
  note: {\bf\_in - wraps up the {\itInflow} block}
      |
      | The init function {\itinit_in} sets up the logging of the level and flow names.
  in : Inport
  back : Inport  Port=2
  Bus Selector : BusSelector  OutputSignals=tau,c,J
  Inflow : $bdroot/Utility/Inflow  SystemSampleTime=-1
  Mux : Mux  Inputs=3
  out : Outport
  wires:
  Bus Selector/2 -> Mux/2  "<c>"
  in/1 -> Inflow/1  "w"
  back/1 -> Bus Selector/1
  Bus Selector/3 -> Mux/3  "<J>"
  Bus Selector/1 -> Mux/1  "<tau>"
  Inflow/1 -> out/1
  Mux/1 -> Inflow/2

== system Simple_lib/Rotational/_out ==
  note: {\bf\_out - buses out and logs the signals from the generic {\itOutflow} block}
      |
      | The init function {\itinit\_out} sets up the logging.
  in : Inport  Tag=NOFLUX
  Bus Creator : BusCreator  Inputs=3
  Constant : Constant  Value=[0;0;0]
  Demux : Demux  Outputs=3
  Outflow : $bdroot/Utility/Outflow  Tag=Electrical  SystemSampleTime=-1
  Sum : Sum  Inputs=|++
  Sum1 : Sum  Inputs=+  CollapseMode=Specified dimension  CollapseDim=2
  out : Outport
  backs : Outport  Tag=NOFLUX  Port=2
  wires:
  Demux/3 -> Bus Creator/3  "J"
  Outflow/1 -> out/1
  Sum1/1 -> Sum/1
  Demux/1 -> Bus Creator/1  "tau"
  Bus Creator/1 -> backs/1
  Outflow/2 -> Sum1/1
  in/1 -> Outflow/1  "w"
  Demux/2 -> Bus Creator/2  "c"
  Constant/1 -> Sum/2
  Sum/1 -> Demux/1

== system Simple_lib/Thermal/CinWall ==
  C : Subsystem  AncestorBlock=PlantUtilityBlockset_lib/Electrical/C  mask{C=wallMass*c_wall}
      mask prompts: C "Capacitance"
      mask Display:
      | color('white')
      | plot([-1 1 1 -1 -1], [-1 -1 1 1 -1])
      | color('black')
      | plot([1.0 1.8 1.8 1.0], [0 .1 -.1 0])
      | plot([-1 -1], [-1 1])
      | plot([1 1], [-1 1])
  Gnd : Subsystem  AncestorBlock=PlantUtilityBlockset_lib/Electrical/Gnd
      mask Display:
      | color('white')
      | plot([-1 1 1 -1 -1], [-1 -1 1 1 -1])
      | 
      | color('black')
      | plot([1.0 1.18 1.18 1.0], [0 .15 -.15 0])
      | 
      | plot([-0.4 -0.4],[-1 1])
      | plot([-0.6 -0.6], [-0.6 0.6])
      | plot([-0.8 -0.8],[-0.2 0.2])
      | 
      | plot([-0.4 1],[0 0])
  Out1 : Outport
  wires:
  C/1(Out1) -> Out1/1
  Gnd/1(Out1) -> C/1(In1)

== system Simple_lib/Thermal/R13 ==
  In1 : Inport
  Duplex : Subsystem  Tag=Electrical  AncestorBlock=PlantUtilityBlockset_lib/Utility/Duplex  InitFcn=initDuplex
      mask Display:
      | color('white')
      | plot([0 3], [2 2])
      | plot([0 3], [-2 -2])
      | color('black')
      | 
      | plot([0 1 1], [0 0 0.4])
      | plot([1 1 3], [0.6 1 1])
      | plot([1 3 2 1 0 2], [0.6 0.6 0.4 0.6 0.4 0.4])
      | patch([0 2 1],[0.4 0.4 0.6],[0,0,0])
      | plot([3 2 2], [1 1 0.6])
      | plot([2 2 3], [0.4 -1 -1])
  Simplex : Subsystem  Tag=Electrical  AncestorBlock=PlantUtilityBlockset_lib/Utility/Simplex  InitFcn=initSimplex
      mask Display:
      | color('white')
      | plot([0 3], [2 2])
      | plot([0 3], [-2 -2])
      | color('black')
      | 
      | plot([0 2 2 3], [1 1 0 0])
      | plot([1 3 2 1 0 2], [0.6 0.6 0.4 0.6 0.4 0.4])
      | patch([1 3 2],[0.6 0.6 0.4],[0,0,0])
      | plot([0 1 1], [1 1 0.6])
      | plot([1 1 0], [0.4 -1 -1])
  Sum : Sum  Inputs=|++
  resistance : Gain  Gain=R
  Out1 : Outport
  wires:
  In1/1 -> Simplex/1(InPot)
  Duplex/1(OutPot) -> Out1/1
  Duplex/2(OutFlow) -> Simplex/2(InFlow), resistance/1
  Simplex/1(OutPot) -> Sum/1
  resistance/1 -> Sum/2
  Sum/1 -> Duplex/1(InPot)

== system Simple_lib/Thermal/R17 ==
  In1 : Inport
  In2 : Inport  Port=2
  1/R1 : Gain  Gain=-1
  1/R2 : Gain  Gain=-1
  Discrete-Time Integrator1 : DiscreteIntegrator  gainval=1/10/Ts  SampleTime=Ts  ICPrevOutput=DiscIntNeverNeededParam  ICPrevScaledInput=DiscIntNeverNeededParam
  Simplex : Subsystem  Tag=Electrical  AncestorBlock=PlantUtilityBlockset_lib/Utility/Simplex  InitFcn=initSimplex
      mask Display:
      | color('white')
      | plot([0 3], [2 2])
      | plot([0 3], [-2 -2])
      | color('black')
      | 
      | plot([0 2 2 3], [1 1 0 0])
      | plot([1 3 2 1 0 2], [0.6 0.6 0.4 0.6 0.4 0.4])
      | patch([1 3 2],[0.6 0.6 0.4],[0,0,0])
      | plot([0 1 1], [1 1 0.6])
      | plot([1 1 0], [0.4 -1 -1])
  Simplex1 : Subsystem  Tag=Electrical  AncestorBlock=PlantUtilityBlockset_lib/Utility/Simplex  InitFcn=initSimplex
      mask Display:
      | color('white')
      | plot([0 3], [2 2])
      | plot([0 3], [-2 -2])
      | color('black')
      | 
      | plot([0 2 2 3], [1 1 0 0])
      | plot([1 3 2 1 0 2], [0.6 0.6 0.4 0.6 0.4 0.4])
      | patch([1 3 2],[0.6 0.6 0.4],[0,0,0])
      | plot([0 1 1], [1 1 0.6])
      | plot([1 1 0], [0.4 -1 -1])
  Sum : Sum  Inputs=+|+
  Sum1 : Sum  Inputs=|+-
  conductance : Gain  Gain=1/R
  wires:
  Discrete-Time Integrator1/1 -> Sum1/2, 1/R1/1, Simplex/2(InFlow)
  Sum1/1 -> Discrete-Time Integrator1/1
  1/R1/1 -> Simplex1/2(InFlow)
  Simplex1/1(OutPot) -> Sum/2
  In2/1 -> Simplex1/1(InPot)
  Sum/1 -> conductance/1
  1/R2/1 -> Sum/1
  Simplex/1(OutPot) -> 1/R2/1
  In1/1 -> Simplex/1(InPot)
  conductance/1 -> Sum1/1

== system Simple_lib/Thermal/ThermoMeter ==
  note: NOTE: Does not necessarily need Pushback
  In : Inport
  Ground : Ground
  PushBack : Subsystem  AncestorBlock=PlantUtilityBlockset_lib/Utility/Push  InitFcn=initSimplex
      mask Display:
      | color('white')
      | plot([0 3], [2 2])
      | plot([0 3], [-2 -2])
      | color('black')
      | 
      | plot([0 2 2 3], [1 1 0 0])
      | plot([1 3 2 1 0 2], [0.6 0.6 0.4 0.6 0.4 0.4])
      | patch([1 3 2],[0.6 0.6 0.4],[0,0,0])
      | plot([0 1 1], [1 1 0.6])
      | plot([1 1 0], [0.4 -1 -1])
  T : Outport
  wires:
  In/1 -> PushBack/1(InPot)
  PushBack/1(OutPot) -> T/1
  Ground/1 -> PushBack/2(InFlow)

== system Simple_lib/Translational/BiGain ==
  In1 : Inport
  Bus Creator1 : BusCreator  Inputs=2
  Bus Selector : BusSelector  OutputSignals=F,M
  _in : $bdroot/Translational/_in  Level=v  Flow=F
  _out : $bdroot/Translational/_out  Tag=Electrical  Level=v  Flow=F
  k_flow : Gain  Gain=k_flow
  k_flow1 : Gain  Gain=k_flow
  k_flow2 : Gain  Gain=k_flow
  k_level : Gain  Gain=k_level
  Out1 : Outport
  wires:
  _out/1 -> Out1/1
  _in/1 -> k_level/1
  In1/1 -> _in/1
  k_level/1 -> _out/1
  _out/2 -> Bus Selector/1
  k_flow/1 -> Bus Creator1/1  "F"
  Bus Selector/2 -> k_flow2/1  "<M>"
  Bus Selector/1 -> k_flow/1  "<F>"
  Bus Creator1/1 -> _in/2
  k_flow2/1 -> k_flow1/1  "M"
  k_flow1/1 -> Bus Creator1/2  "M"

== system Simple_lib/Translational/Damping ==
  + : Inport
  - : Inport  Port=2
  1/R3 : Gain  Gain=b
  Bus Creator : BusCreator  Inputs=2
  Bus Creator1 : BusCreator  Inputs=2
  Gain1 : Gain  Gain=-1
  Ground : Ground
  Ground1 : Ground
  Sum : Sum  Inputs=+|-
  _neg : $bdroot/Translational/_in  Level=v  Flow=F
  _pos : $bdroot/Translational/_in  Level=v  Flow=F
  wires:
  _neg/1 -> Sum/2
  1/R3/1 -> Bus Creator/1, Gain1/1  "F"
  Bus Creator1/1 -> _pos/2
  Ground/1 -> Bus Creator/2  "M"
  +/1 -> _pos/1
  _pos/1 -> Sum/1
  Sum/1 -> 1/R3/1
  -/1 -> _neg/1
  Bus Creator/1 -> _neg/2
  Ground1/1 -> Bus Creator1/2  "M"
  Gain1/1 -> Bus Creator1/1  "F"

== system Simple_lib/Translational/Friction ==
  pos : Inport
  K : Inport  Port=2
  neg : Inport  Port=3
  1/R1 : Gain  Gain=-1
  1/R2 : Gain  Gain=-1
  1/R3 : Gain  Gain=-1
  Bus Creator : BusCreator  Inputs=2
  Bus Creator1 : BusCreator  Inputs=2
  Discrete-Time Integrator : DiscreteIntegrator  gainval=1  SampleTime=-1  ICPrevOutput=DiscIntNeverNeededParam  ICPrevScaledInput=DiscIntNeverNeededParam
  Exp : Math  SaturateOnIntegerOverflow=on
  Gain : Gain  Gain=-1/2
  Ground : Ground
  Multiply : Product
  Multiply1 : Product  Inputs=**//
  Multiply2 : Product  Inputs=**/
  Sum : Sum  Inputs=+|+
  Sum1 : Sum  Inputs=|++
  _neg : $bdroot/Translational/_in  Level=v  Flow=F
  _pos : $bdroot/Translational/_in  Level=v  Flow=F
  friction : Trigonometry  Operator=tanh
  grab : Gain  Gain=grab
  sigma : Constant  Value=s
  synche : Gain  Gain=Ki/sqrt(2*pi)
  wires:
  synche/1 -> Sum1/2
  friction/1 -> Multiply/2
  Sum/1 -> grab/1
  Discrete-Time Integrator/1 -> synche/1
  Sum1/1 -> friction/1
  Gain/1 -> Exp/1
  sigma/1 -> Multiply1/3, Multiply1/4, Multiply2/3
  Multiply2/1 -> Discrete-Time Integrator/1
  Exp/1 -> Multiply2/2
  Multiply1/1 -> Gain/1
  _neg/1 -> 1/R3/1
  Multiply/1 -> 1/R2/1
  _pos/1 -> Sum/1
  grab/1 -> Multiply2/1, Multiply1/2, Multiply1/1, Sum1/1
  pos/1 -> _pos/1
  neg/1 -> _neg/1
  K/1 -> Multiply/1
  Bus Creator1/1 -> _pos/2
  1/R2/1 -> Bus Creator1/1, 1/R1/1  "F"
  Bus Creator/1 -> _neg/2
  Ground/1 -> Bus Creator1/2, Bus Creator/2  "M"
  1/R1/1 -> Bus Creator/1  "F"
  1/R3/1 -> Sum/2

== system Simple_lib/Translational/Sink ==
  In1 : Inport
  Bus Creator : BusCreator  Inputs=2
  Constant : Constant  Value=m
  Ground : Ground
  Terminator : Terminator
  _at : $bdroot/Translational/_in  Level=v  Flow=F
  wires:
  Bus Creator/1 -> _at/2
  In1/1 -> _at/1
  _at/1 -> Terminator/1
  Ground/1 -> Bus Creator/1  "F"
  Constant/1 -> Bus Creator/2  "M"

== system Simple_lib/Translational/Source ==
  note: Newton's law for all the applied torques (real parts) and the inertials (imaginary parts).
  Bus Selector : BusSelector  OutputSignals=F,M
  Constant : Constant  Value=m
  Discrete-Time Integrator1 : DiscreteIntegrator  gainval=1  InitialCondition=v_0  SampleTime=-1  ICPrevOutput=DiscIntNeverNeededParam  ICPrevScaledInput=DiscIntNeverNeededParam
  Multiply : Product  Inputs=*/
  Saturation : Saturate  UpperLimit=inf  LowerLimit=Ts*1e-3
  Sum : Sum  Inputs=|++
  _at : $bdroot/Translational/_out  Tag=Electrical  Level=v  Flow=F
  Out1 : Outport
  wires:
  _at/1 -> Out1/1
  Multiply/1 -> Discrete-Time Integrator1/1
  _at/2 -> Bus Selector/1
  Bus Selector/1 -> Multiply/1  "<F>"
  Bus Selector/2 -> Sum/1  "<M>"
  Sum/1 -> Saturation/1
  Constant/1 -> Sum/2
  Discrete-Time Integrator1/1 -> _at/1
  Saturation/1 -> Multiply/2

== system Simple_lib/Translational/SpringDamper ==
  in : Inport
  Damping : $bdroot/Translational/Damping  b=b_damper
  Source1 : $bdroot/Translational/Source  m=m_out  v_0=v_0
      settings: AttributesFormatString=%<m> kg
  Stiffness : $bdroot/Translational/Stiffness  k_spring=k_spring  s_0=s_0  I_spring=m_split  b_series=b_spring
  Terminator : Terminator
  out : Outport
  wires:
  in/1 -> Damping/1, Stiffness/1
  Source1/1 -> Damping/2, Stiffness/2, out/1
  Stiffness/1 -> Terminator/1

== system Simple_lib/Translational/Stiffness ==
  + : Inport
  - : Inport  Port=2
  Bus Creator : BusCreator  Inputs=2
  Bus Creator1 : BusCreator  Inputs=2
  Constant : Constant  Value=I_spring/2
  Constant1 : Constant  Value=I_spring/2
  Discrete-Time Integrator1 : DiscreteIntegrator  gainval=1  InitialCondition=s_0  SampleTime=-1  ICPrevOutput=DiscIntNeverNeededParam  ICPrevScaledInput=DiscIntNeverNeededParam
  Gain : Gain  Gain=-k_spring
  Gain1 : Gain  Gain=k_spring
  Gain2 : Gain  Gain=2/b_series
  Gain3 : Gain  Gain=2/b_series
  Sum : Sum  Inputs=+|-
  Sum1 : Sum  Inputs=++|
  Sum2 : Sum  Inputs=++|
  _neg : $bdroot/Translational/_in  Level=v  Flow=F
  _pos : $bdroot/Translational/_in  Level=v  Flow=F
  cmp : Outport
  wires:
  _neg/1 -> Sum2/1
  -/1 -> _neg/1
  Sum/1 -> Discrete-Time Integrator1/1
  _pos/1 -> Sum1/1
  +/1 -> _pos/1
  Bus Creator1/1 -> _pos/2
  Bus Creator/1 -> _neg/2
  Discrete-Time Integrator1/1 -> cmp/1, Gain1/1, Gain/1  "cmp"
  Constant/1 -> Bus Creator1/2  "M"
  Constant1/1 -> Bus Creator/1  "M"
  Sum2/1 -> Sum/2
  Sum1/1 -> Sum/1
  Gain/1 -> Gain2/1, Bus Creator1/1  "F"
  Gain1/1 -> Bus Creator/2, Gain3/1  "F"
  Gain2/1 -> Sum1/2
  Gain3/1 -> Sum2/2

== system Simple_lib/Translational/_in ==
  note: {\bf\_in - wraps up the {\itInflow} block}
      |
      | The init function {\itinit_in} sets up the logging of the level and flow names.
  in : Inport
  back : Inport  Port=2
  Bus Selector : BusSelector  OutputSignals=F,M
  Inflow : $bdroot/Utility/Inflow  SystemSampleTime=-1
  Mux : Mux  Inputs=2
  out : Outport
  wires:
  in/1 -> Inflow/1  "v"
  back/1 -> Bus Selector/1
  Bus Selector/2 -> Mux/2  "<M>"
  Bus Selector/1 -> Mux/1  "<F>"
  Inflow/1 -> out/1
  Mux/1 -> Inflow/2

== system Simple_lib/Translational/_out ==
  note: {\bf\_out - buses out and logs the signals from the generic {\itOutflow} block}
      |
      | The init function {\itinit\_out} sets up the logging.
  in : Inport  Tag=NOFLUX
  Bus Creator : BusCreator  Inputs=2
  Constant : Constant  Value=[0;0]
  Demux : Demux  Outputs=2
  Outflow : $bdroot/Utility/Outflow  Tag=Electrical  SystemSampleTime=-1
  Sum : Sum  Inputs=|++
  Sum1 : Sum  Inputs=+  CollapseMode=Specified dimension  CollapseDim=2
  out : Outport
  backs : Outport  Tag=NOFLUX  Port=2
  wires:
  Outflow/1 -> out/1
  Sum1/1 -> Sum/1
  Demux/1 -> Bus Creator/1  "F"
  Bus Creator/1 -> backs/1
  Outflow/2 -> Sum1/1
  in/1 -> Outflow/1  "v"
  Demux/2 -> Bus Creator/2  "M"
  Constant/1 -> Sum/2
  Sum/1 -> Demux/1

== system Simple_lib/Utility/BiGain ==
  In1 : Inport
  Duplex : $bdroot/Utility/Outflow  Tag=Electrical  SystemSampleTime=-1
  Simplex : $bdroot/Utility/Inflow  Tag=Electrical  SystemSampleTime=-1
  Sum1 : Sum  Inputs=+
  k_flow : Gain  Gain=k_flow
  k_pot : Gain  Gain=k_pot
  Out1 : Outport
  wires:
  Duplex/2 -> Sum1/1
  Duplex/1 -> Out1/1
  Simplex/1 -> k_pot/1
  In1/1 -> Simplex/1
  k_flow/1 -> Simplex/2
  k_pot/1 -> Duplex/1
  Sum1/1 -> k_flow/1

== system Simple_lib/Utility/Duplex ==
  InPot : Inport  Tag=NOFLUX
  FlowGain : Gain
  FlowSum : Sum  Inputs=3  SaturateOnIntegerOverflow=on  InputSameDT=on  OutDataTypeStr=Inherit: Same as first input
  OutPot : Outport
  OutFlow : Outport  Tag=NOFLUX  Port=2
  wires:
  [SimplexR1StatorHeatSinkInverterPFessSchematicPower] -> FlowSum/3
  [SimplexR2StatorHeatSinkInverterPFessSchematicPower] -> FlowSum/2
  [SimplexR3StatorHeatSinkInverterPFessSchematicPower] -> FlowSum/1
  FlowGain/1 -> OutFlow/1  "flow"
  InPot/1 -> OutPot/1  "pot"
  FlowSum/1 -> FlowGain/1

== system Simple_lib/Utility/DuplexSav ==
  InPot : Inport  Tag=NOFLUX
  FlowDisplay : Display
  FlowGain : Gain
  Flow_DuplexGndC0ChargingCapacitor3 : Scope
      settings: Tag=Flow
  PotDisplay : Display
  Pot_DuplexGndC0ChargingCapacitor3 : Scope
      settings: Tag=Pot
  Rate Transition : RateTransition  OutPortSampleTimeMultiple=nT  OutPortSampleTime=Ts
  OutPot : Outport
  OutFlow : Outport  Tag=NOFLUX  Port=2
  wires:
  [SimplexCC0ChargingCapacitor3] -> FlowGain/1
  FlowGain/1 -> FlowDisplay/1, OutFlow/1, Flow_DuplexGndC0ChargingCapacitor3/1
  InPot/1 -> Pot_DuplexGndC0ChargingCapacitor3/1, PotDisplay/1, Rate Transition/1
  Rate Transition/1 -> OutPot/1

== system Simple_lib/Utility/Inflow ==
  note: {\bfBack - sends a signal back using a {\itGoto} block}
      |
      | The init function {\itsmpInit} creates the Goto block with a unique name.
  in : Inport
  back : Inport  Port=2
  Terminator : Terminator
  out : Outport
  tag scope: tagInflowUtilitySimple_lib=global
  wires:
  back/1 -> [tagInflowUtilitySimple_lib]
  in/1 -> out/1
  [tagInflowUtilitySimple_lib] -> Terminator/1

== system Simple_lib/Utility/Inflow_old ==
  note: {\bfBack - sends a signal back using a {\itGoto} block}
      |
      | The init function {\itinitBack} creates the Goto block with a unique name.
  in : Inport
  back : Inport  Tag=NOFLUX  Port=2
  out : Outport
  tag scope: tagInflow_oldUtilitySimple_lib=global
  wires:
  back/1 -> [tagInflow_oldUtilitySimple_lib]  "FlowInflowUtilityLumped_lib"
  in/1 -> out/1  "LevelInflowUtilityLumped_lib"

== system Simple_lib/Utility/Inflow_old1 ==
  note: {\bfBack - sends a signal back using a {\itGoto} block}
      |
      | The init function {\itinitBack} creates the Goto block with a unique name.
  in : Inport
  back : Inport  Tag=NOFLUX  Port=2
  out : Outport
  tag scope: tagInflow_old1UtilitySimple_lib=global
  wires:
  back/1 -> [tagInflow_old1UtilitySimple_lib]  "FlowInflowUtilityLumped_lib"
  in/1 -> out/1  "LevelInflowUtilityLumped_lib"

== system Simple_lib/Utility/Outflow ==
  note: {\bfOutput - buses out all the back signals sent by {\itGoto} blocks}
      |
      | The init function {\itinitOutput} creates the From blocks and links them to BackBus
  in : Inport  Tag=NOFLUX
  BackBus : Concatenate  NumInputs=1  Mode=Multidimensional array  ConcatenateDimension=2
  out : Outport
  backs : Outport  Tag=NOFLUX  Port=2
  wires:
  BackBus/1 -> backs/1
  in/1 -> out/1

== system Simple_lib/Utility/Outflow_old ==
  note: {\bfOutput - buses out all the back signals sent by {\itGoto} blocks}
      |
      | The init function {\itinitOutput} creates the From blocks and links them to BackBus
  in : Inport  Tag=NOFLUX
  BackBus : BusCreator  Inputs=1
  out : Outport
  backs : Outport  Tag=NOFLUX  Port=2
  wires:
  BackBus/1 -> backs/1  "Flows"
  in/1 -> out/1  "Level"

== system Simple_lib/Utility/Outflow_old1 ==
  note: {\bfOutput - buses out all the back signals sent by {\itGoto} blocks}
      |
      | The init function {\itinitOutput} creates the From blocks and links them to BackBus
  in : Inport  Tag=NOFLUX
  BackBus : BusCreator  Inputs=1
  out : Outport
  backs : Outport  Tag=NOFLUX  Port=2
  wires:
  in/1 -> out/1  "Level"
  BackBus/1 -> backs/1  "Flows"

== system Simple_lib/Utility/Pull ==
  InPot : Inport  Tag=NOFLUX
  FlowGain : Gain
  FlowSum : Sum  Inputs=4  SaturateOnIntegerOverflow=on  InputSameDT=on  OutDataTypeStr=Inherit: Same as first input
  OutPot : Outport
  OutFlow : Outport  Tag=NOFLUX  Port=2
  wires:
  InPot/1 -> OutPot/1  "p_DuplexInverter_test0"
  FlowGain/1 -> OutFlow/1  "f_DuplexInverter_test0"
  FlowSum/1 -> FlowGain/1
  [Push_inSynchroGearsR1_6HYBPTPlantHYBPT_test] -> FlowSum/1
  [Push_inSynchro4GearsR1_6HYBPTPlantHYBPT_test] -> FlowSum/2
  [Push_inSynchro2GearsR1_6HYBPTPlantHYBPT_test] -> FlowSum/3
  [Push_inSynchro1GearsR1_6HYBPTPlantHYBPT_test] -> FlowSum/4

== system Simple_lib/Utility/Push ==
  InPot : Inport
  InFlow : Inport  Tag=NOFLUX  Port=2
  OutPot : Outport  Tag=NOFLUX
  tag scope: Push_inSynchro5GearsR1_6HYBPTPlantHYBPT_test=global
  wires:
  InFlow/1 -> [Push_inSynchro5GearsR1_6HYBPTPlantHYBPT_test]  "flow"
  InPot/1 -> OutPot/1  "pot"

== system Simple_lib/Utility/Simplex ==
  InPot : Inport
  InFlow : Inport  Tag=NOFLUX  Port=2
  OutPot : Outport  Tag=NOFLUX
  tag scope: SimplexCThermalInertiaInverterPFessSchematicPower=global
  wires:
  InFlow/1 -> [SimplexCThermalInertiaInverterPFessSchematicPower]  "flow"
  InPot/1 -> OutPot/1  "pot"
